simulink model "zbiornik2"  (R2015a)
settings: Solver=ode3  StartTime=0.0  StopTime=50  FixedStep=0.01  RelTol=1e-3
values from neighbouring files (symbols this model uses):
  a2 = x1(2)    [ident1.m]    (also in wyniki_akt.mat = 0.5)
  b = 37    [ident1.m]    (also in wyniki_akt.mat; zbiornik_1.m; zbiornik_2.m; zbiornik_3.m)
  c = 10    [ident1.m]    (also in wyniki_akt.mat; zbiornik_1.m; zbiornik_2.m; zbiornik_3.m)
  C2 = x1(1)    [ident1.m]    (also in wyniki_akt.mat = 30)
  h20 = max(y2)    [ucinanie.m]
  h2max = 35    [ident1.m]    (also in wyniki_akt.mat; zbiornik_1.m; zbiornik_2.m; zbiornik_3.m)
  w = 5    [ident1.m]    (also in wyniki_akt.mat; zbiornik_1.m; zbiornik_2.m; zbiornik_3.m)
settings Model: Creator=Ziger  LastModifiedBy=Student

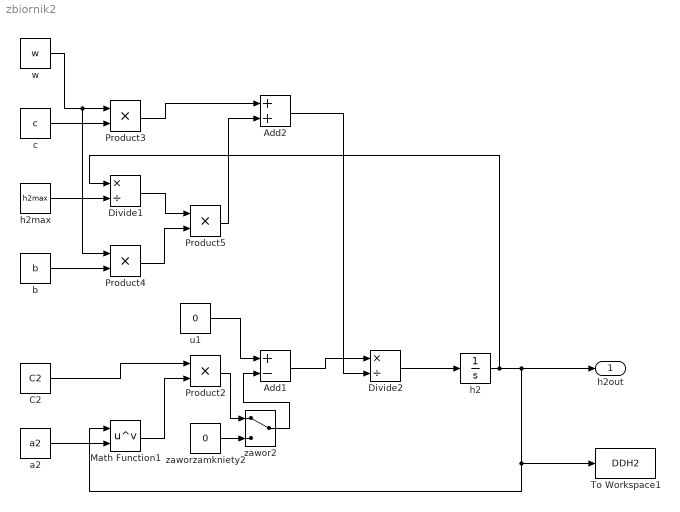
== system zbiornik2 ==
  Add1 : Sum  Inputs=+-
  Add2 : Sum
  C2 : Constant  Value=C2
  Divide1 : Product  Inputs=*/
  Divide2 : Product  Inputs=*/
  Math Function1 : Math  Operator=pow  SaturateOnIntegerOverflow=on
  Product{2..5} (4 alike) : Product
  To Workspace1 : ToWorkspace  VariableName=DDH2  SaveFormat=Structure With Time  SampleTime=-1
  a2 : Constant  Value=a2
  b : Constant  Value=b
  c : Constant  Value=c
  h2 : Integrator  InitialCondition=h20  LimitOutput=on  UpperSaturationLimit=35  LowerSaturationLimit=0
  h2max : Constant  Value=h2max
  u1 : Constant  Value=0
  w : Constant  Value=w
  "zawor2 " : ManualSwitch
  zaworzamkniety2 : Constant  Value=0
  "h2out " : Outport
  wires:
  h2/1 -> Divide1/1, "h2out "/1, To Workspace1/1, Math Function1/1
  Math Function1/1 -> Product2/2
  Product4/1 -> Product5/2
  h2max/1 -> Divide1/2
  C2/1 -> Product2/1
  w/1 -> Product4/1, Product3/1
  Divide2/1 -> h2/1
  Add2/1 -> Divide2/2
  Divide1/1 -> Product5/1
  a2/1 -> Math Function1/2
  Product5/1 -> Add2/2
  b/1 -> Product4/2
  Product3/1 -> Add2/1
  Add1/1 -> Divide2/1
  c/1 -> Product3/2
  Product2/1 -> "zawor2 "/1
  zaworzamkniety2/1 -> "zawor2 "/2
  "zawor2 "/1 -> Add1/2
  u1/1 -> Add1/1
